simulink model "hardcode_testing_with_rate_adaptive"  (R2020b)
settings: Solver=FixedStepAuto  StartTime=0.0  StopTime=30  FixedStep=1E-3  RelTol=1e-3  EnableMultiTasking=on
undefined symbols (not defined in the file): D0, D1, D10, D11, D12, D13, D2, D3, D4, D5, D6, D7, D8, D9, PTA0, PTA1, PTA2, PTB23, PTB9, PTC16, PTC17, PTC2, PTC3, PTC4, PTD0, PTD1, PTD2, PTD3
libraries: frdmk64flib x17
settings Model: SimulationMode=external  ExtModeTrigDuration=5  Creator=Owner  LastModifiedBy=saihajgill
settings OptimizationCC: EnhancedBackFolding=on  PassReuseOutputArgsAs=Individual arguments  ZeroExternalMemoryAtStartup=off  ZeroInternalMemoryAtStartup=off  MaxStackSize=64  OptimizeBlockOrder=speed  DifferentSizesBufferReuse=on  OptimizationCustomize=off  EfficientTunableParamExpr=on
settings DebuggingCC: ParameterTunabilityLossMsg=error
settings HardwareCC: ProdBitPerPointer=32  ProdBitPerSizeT=32  ProdBitPerPtrDiffT=32  ProdLargestAtomicInteger=Long  ProdLargestAtomicFloat=Double  ProdWordSize=32  ProdHWDeviceType=ARM Compatible->ARM Cortex  UseEmbeddedCoderFeatures=off
settings SFSimCC: MATLABDynamicMemAlloc=off
settings RTWCC: Description=Embedded Coder  SystemTargetFile=ert.tlc  HardwareBoard=NXP FRDM-K64F  TLCOptions="-aInlineSetEventsForThisBaseRateFcn=TLC_FALSE -aSuppressMultiTaskScheduler=TLC_FALSE  -aRateBasedStepFcn=0"  TemplateMakefile=ert_default_tmf  Toolchain=GNU Tools for ARM Embedded Processors
settings CodeAppCC: ForceParamTrailComments=on  IgnoreCustomStorageClasses=off  OperatorAnnotations=on  SimulinkDataObjDesc=on  SFDataObjDesc=on  InsertBlockDesc=on
settings ERTTargetCC: SupportNonInlinedSFcns=on  ExtModeTransport=4  ExtModeMexFile=sendToCommService

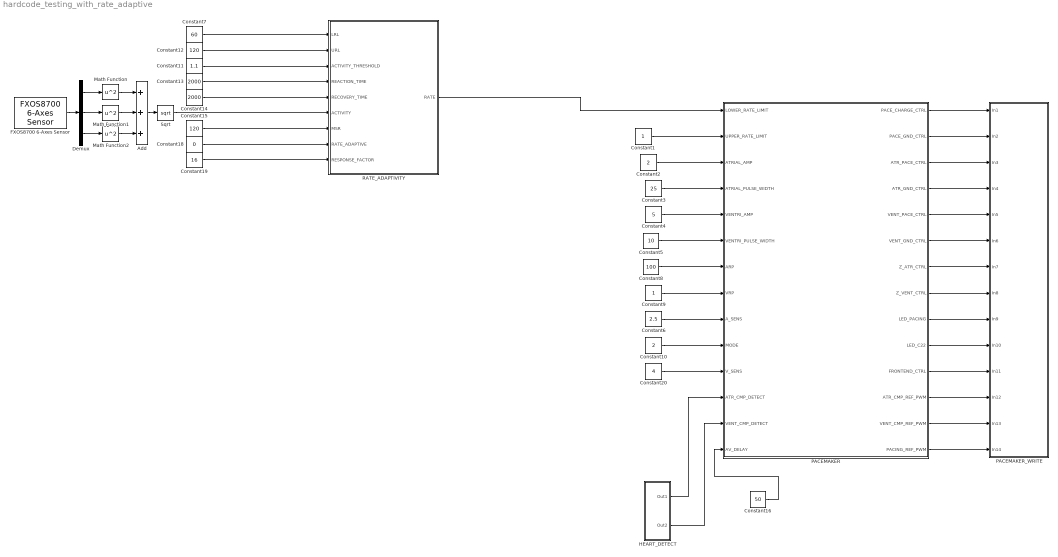
== system hardcode_testing_with_rate_adaptive ==
  Add : Sum  Inputs=+++
  Constant1 : Constant
  Constant10 : Constant  Value=2
  Constant11 : Constant  Value=1.1
  Constant12 : Constant  Value=120
  Constant13 : Constant  Value=2000
  Constant14 : Constant  Value=2000
  Constant15 : Constant  Value=120
  Constant16 : Constant  Value=50
  Constant18 : Constant  Value=0
  Constant19 : Constant  Value=16
  Constant2 : Constant  Value=2
  Constant20 : Constant  Value=4
  Constant3 : Constant  Value=25
  Constant4 : Constant  Value=5
  Constant5 : Constant  Value=10
  Constant6 : Constant  Value=2.5
  Constant7 : Constant  Value=60
  Constant8 : Constant  Value=100
  Constant9 : Constant
  Demux : Demux  Outputs=3
  FXOS8700 6-Axes Sensor : frdmk64flib/FXOS8700 6-Axes Sensor  Activesensor=Accelerometer only  ODR=800Hz  HybridODR=400Hz  Accelfullrange=-4g to +4g  SampleTime=-1
  HEART_DETECT : Subsystem
  Math Function : Math  Operator=square  SaturateOnIntegerOverflow=on
  Math Function1 : Math  Operator=square  SaturateOnIntegerOverflow=on
  Math Function2 : Math  Operator=square  SaturateOnIntegerOverflow=on
  PACEMAKER : Stateflow chart  TreatAsAtomicUnit=on
  PACEMAKER_WRITE : Subsystem
  RATE_ADAPTIVITY : Stateflow chart  TreatAsAtomicUnit=on
  Sqrt : Sqrt  SaturateOnIntegerOverflow=on
  wires:
  Constant1/1 -> PACEMAKER/2(UPPER_RATE_LIMIT)
  Constant2/1 -> PACEMAKER/3(ATRIAL_AMP)
  Constant3/1 -> PACEMAKER/4(ATRIAL_PULSE_WIDTH)
  Constant4/1 -> PACEMAKER/5(VENTRI_AMP)
  Constant5/1 -> PACEMAKER/6(VENTRI_PULSE_WIDTH)
  Constant8/1 -> PACEMAKER/7(ARP)
  Constant9/1 -> PACEMAKER/8(VRP)
  Constant10/1 -> PACEMAKER/10(MODE)
  Constant6/1 -> PACEMAKER/9(A_SENS)
  PACEMAKER/1(PACE_CHARGE_CTRL) -> PACEMAKER_WRITE/1(In1)
  PACEMAKER/2(PACE_GND_CTRL) -> PACEMAKER_WRITE/2(In2)
  PACEMAKER/3(ATR_PACE_CTRL) -> PACEMAKER_WRITE/3(In3)
  PACEMAKER/4(ATR_GND_CTRL) -> PACEMAKER_WRITE/4(In4)
  PACEMAKER/5(VENT_PACE_CTRL) -> PACEMAKER_WRITE/5(In5)
  PACEMAKER/6(VENT_GND_CTRL) -> PACEMAKER_WRITE/6(In6)
  PACEMAKER/7(Z_ATR_CTRL) -> PACEMAKER_WRITE/7(In7)
  PACEMAKER/8(Z_VENT_CTRL) -> PACEMAKER_WRITE/8(In8)
  PACEMAKER/9(LED_PACING) -> PACEMAKER_WRITE/9(In9)
  PACEMAKER/10(LED_C22) -> PACEMAKER_WRITE/10(In10)
  PACEMAKER/11(FRONTEND_CTRL) -> PACEMAKER_WRITE/11(In11)
  PACEMAKER/12(ATR_CMP_REF_PWM) -> PACEMAKER_WRITE/12(In12)
  PACEMAKER/13(VENT_CMP_REF_PWM) -> PACEMAKER_WRITE/13(In13)
  PACEMAKER/14(PACING_REF_PWM) -> PACEMAKER_WRITE/14(In14)
  HEART_DETECT/1(Out1) -> PACEMAKER/12(ATR_CMP_DETECT)
  HEART_DETECT/2(Out2) -> PACEMAKER/13(VENT_CMP_DETECT)
  Demux/2 -> Math Function1/1
  Constant15/1 -> RATE_ADAPTIVITY/7(MSR)
  Constant12/1 -> RATE_ADAPTIVITY/2(URL)
  Constant19/1 -> RATE_ADAPTIVITY/9(RESPONSE_FACTOR)
  Add/1 -> Sqrt/1
  Demux/3 -> Math Function2/1
  Constant13/1 -> RATE_ADAPTIVITY/4(REACTION_TIME)
  Constant18/1 -> RATE_ADAPTIVITY/8(RATE_ADAPTIVE)
  FXOS8700 6-Axes Sensor/1 -> Demux/1
  Math Function1/1 -> Add/2
  Constant14/1 -> RATE_ADAPTIVITY/5(RECOVERY_TIME)
  Demux/1 -> Math Function/1
  Constant7/1 -> RATE_ADAPTIVITY/1(LRL)
  Math Function2/1 -> Add/3
  Constant11/1 -> RATE_ADAPTIVITY/3(ACTIVITY_THRESHOLD)
  Math Function/1 -> Add/1
  Sqrt/1 -> RATE_ADAPTIVITY/6(ACTIVITY)
  Constant16/1 -> PACEMAKER/14(AV_DELAY)
  Constant20/1 -> PACEMAKER/11(V_SENS)
  RATE_ADAPTIVITY/1(RATE) -> PACEMAKER/1(LOWER_RATE_LIMIT)

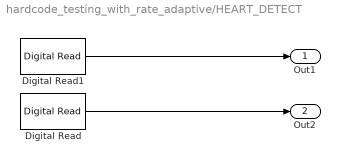
== system hardcode_testing_with_rate_adaptive/HEART_DETECT ==
  Digital Read : frdmk64flib/Digital Read  Whichpin=PTC17 (D1)  SampleTime=-1
  Digital Read1 : frdmk64flib/Digital Read  Whichpin=PTC16 (D0)  SampleTime=-1
  Out1 : Outport
  Out2 : Outport  Port=2
  wires:
  Digital Read/1 -> Out2/1
  Digital Read1/1 -> Out1/1

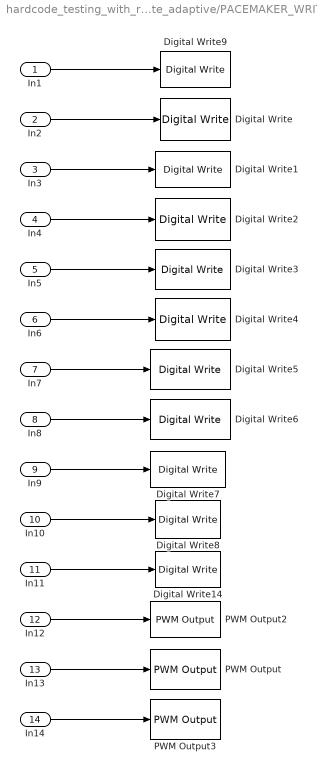
== system hardcode_testing_with_rate_adaptive/PACEMAKER_WRITE ==
  In1 : Inport
  In2 : Inport  Port=2
  In3 : Inport  Port=3
  In4 : Inport  Port=4
  In5 : Inport  Port=5
  In6 : Inport  Port=6
  In7 : Inport  Port=7
  In8 : Inport  Port=8
  In9 : Inport  Port=9
  In10 : Inport  Port=10
  In11 : Inport  Port=11
  In12 : Inport  Port=12
  In13 : Inport  Port=13
  In14 : Inport  Port=14
  Digital Write : frdmk64flib/Digital Write  Whichpin=PTD0 (D10)
  Digital Write1 : frdmk64flib/Digital Write  Whichpin=PTA0 (D8)
  Digital Write14 : frdmk64flib/Digital Write  Whichpin=PTD1 (D13)
  Digital Write2 : frdmk64flib/Digital Write  Whichpin=PTD2 (D11)
  Digital Write3 : frdmk64flib/Digital Write  Whichpin=PTC4 (D9)
  Digital Write4 : frdmk64flib/Digital Write  Whichpin=PTD3 (D12)
  Digital Write5 : frdmk64flib/Digital Write  Whichpin=PTB23 (D4)
  Digital Write6 : frdmk64flib/Digital Write  Whichpin=PTC3 (D7)
  Digital Write7 : frdmk64flib/Digital Write  Whichpin=RED_LED
  Digital Write8 : frdmk64flib/Digital Write  Whichpin=BLUE_LED
  Digital Write9 : frdmk64flib/Digital Write  Whichpin=PTB9 (D2)
  PWM Output : frdmk64flib/PWM Output  Whichpin=PTA1 (D3)  InitialFrequency=2000  InitialDutyCycle=100
  PWM Output2 : frdmk64flib/PWM Output  Whichpin=PTC2 (D6)  InitialFrequency=2000  InitialDutyCycle=100
  PWM Output3 : frdmk64flib/PWM Output  Whichpin=PTA2 (D5)  InitialFrequency=2000  InitialDutyCycle=100
  wires:
  In10/1 -> Digital Write8/1
  In2/1 -> Digital Write/1
  In12/1 -> PWM Output2/1
  In7/1 -> Digital Write5/1
  In4/1 -> Digital Write2/1
  In8/1 -> Digital Write6/1
  In11/1 -> Digital Write14/1
  In1/1 -> Digital Write9/1
  In6/1 -> Digital Write4/1
  In9/1 -> Digital Write7/1
  In14/1 -> PWM Output3/1
  In3/1 -> Digital Write1/1
  In13/1 -> PWM Output/1
  In5/1 -> Digital Write3/1

== stateflow chart hardcode_testing_with_rate_adaptive/RATE_ADAPTIVITY ==
  state BELOW_THRESHOLD [commented out]
    ADJUSTED_BPM = LRL
  state DEFAULT [commented out]
  state ADJUSTED_BPM [commented out]
    entry:
    ADJUSTED_BPM = 13/RESPONSE_FACTOR*(ACTIVITY- ACTIVITY_THRESHOLD)+LRL
  state INIT1 [commented out]
    AVG_ACCEL = 0
    n = 0
  state MIN_RATE
    AVG_ACTIVITY = (AVG_ACTIVITY + ACTIVITY)/2
    if RATE > LRL
    RATE = RATE - (MSR-LRL)/RECOVERY_TIME
    DELAY = RECOVERY_TIME
    else
    RATE = LRL
    DELAY = 0
    end
  state TRANSITION [commented out]
  state INITIAL
    RATE = LRL
    AVG_ACTIVITY = ACTIVITY
  state RATE_ADAPTIVE_DEFAULT
  state RATE_ADAPTIVE
    ADJUSTED_RATE = (0.57*RESPONSE_FACTOR^2-1.34*RESPONSE_FACTOR+22.71)*(AVG_ACTIVITY- double(ACTIVITY_THRESHOLD))+LRL
    if ADJUSTED_RATE > MSR
    ADJUSTED_RATE = MSR
    elseif ADJUSTED_RATE < LRL
    ADJUSTED_RATE = LRL
    end
  state OFFSET
    AVG_ACTIVITY = (AVG_ACTIVITY + ACTIVITY)/2
    if RATE > ADJUSTED_RATE
    RATE = RATE - (MSR-LRL)/RECOVERY_TIME
    DELAY = RECOVERY_TIME
    elseif RATE < ADJUSTED_RATE
    RATE = RATE + (MSR-LRL)/REACTION_TIME
    DELAY = REACTION_TIME
    end
  state INIT [commented out]
    ADJUSTED_BPM = LRL
  state MIN_BPM [commented out]
    ADJUSTED_BPM = LRL
  state SAME_BPM [commented out]
    %no change in bpm
  state UP_BPM [commented out]
    ADJUSTED_BPM =ADJUSTED_BPM + OFFSET
  state MAX_BPM [commented out]
    ADJUSTED_BPM = URL
  state DOWN_BPM [commented out]
    ADJUSTED_BPM = ADJUSTED_BPM - OFFSET
  DEFAULT -> BELOW_THRESHOLD [commented out] : [n>= REACTION_TIME && AVG_ACCEL <= ACTIVITY_THRESHOLD]
  BELOW_THRESHOLD -> DEFAULT [commented out] : {n=1}
  DEFAULT -> DEFAULT [commented out] : [after(1,msec)]{n = n+1, PREV_ACCEL = AVG_ACCEL, AVG_ACCEL = (AVG_ACCEL + CURR_ACCEL)/2}
  (default) -> INIT1 [commented out]
  DEFAULT -> ADJUSTED_BPM [commented out] : [n>= REACTION_TIME && AVG_ACCEL > PREV_ACCEL && AVG_ACCEL >ACTIVITY_THRESHOLD]
  INIT1 -> DEFAULT [commented out]
  DEFAULT -> ADJUSTED_BPM [commented out] : [n>= RECOVERY_TIME && AVG_ACCEL < PREV_ACCEL && AVG_ACCEL > ACTIVITY_THRESHOLD]
  ADJUSTED_BPM -> TRANSITION [commented out] : {n=1}
  TRANSITION -> DEFAULT [commented out] : [BPM >= URL]{BPM = URL, BPM_PREV = BPM}
  TRANSITION -> DEFAULT [commented out] : [BPM >= MSR]{BPM = MSR, BPM_PREV = BPM}
  MIN_RATE -> RATE_ADAPTIVE [order 1] : [n>= DELAY && AVG_ACTIVITY>=ACTIVITY_THRESHOLD]
  MIN_RATE -> MIN_RATE [order 2] : after(1,msec){n=n+1}
  MIN_RATE -> INITIAL [order 3] : [RATE_ADAPTIVE == 0 && n>=DELAY]
  RATE_ADAPTIVE_DEFAULT -> MIN_RATE [order 2] : [AVG_ACTIVITY < ACTIVITY_THRESHOLD]{n=0}
  (default) -> INITIAL
  INITIAL -> RATE_ADAPTIVE_DEFAULT : [RATE_ADAPTIVE == 1]{ADJUSTED_RATE = RATE}
  RATE_ADAPTIVE_DEFAULT -> RATE_ADAPTIVE [order 1] : [AVG_ACTIVITY>= ACTIVITY_THRESHOLD]
  OFFSET -> RATE_ADAPTIVE_DEFAULT [order 1] : [n>=DELAY]
  RATE_ADAPTIVE -> OFFSET : {n=0, AVG_ACTIVITY = ACTIVITY}
  UP_BPM -> SAME_BPM [commented out] : [RATE_ADAPTIVITY == 1 && CUR_ACCEL < ACTIVITY_THRESHOLD && after(REACTION_TIME, msec)]
  OFFSET -> OFFSET [order 2] : after(1, msec){n=n+1}
  MIN_BPM -> UP_BPM [commented out] : [RATE_ADAPTIVITY == 1 && CUR_ACCEL >= ACTIVITY_THRESHOLD && after(REACTION_TIME, msec)]
  (default) -> INIT [commented out]
  SAME_BPM -> UP_BPM [commented out] : [RATE_ADAPTIVITY == 1 &&CUR_ACCEL >= ACTIVITY_THRESHOLD && after(ADJUSTED_BPM, msec)]
  INIT -> MIN_BPM [commented out] : [RATE_ADAPTIVITY == 1]{OFFSET = (MSR-LRL)/RESPONSE_FACTOR}
  DOWN_BPM -> MIN_BPM [commented out] : [RATE_ADAPTIVITY == 0 && after(RECOVERY_TIME, msec) && ADJUSTED_BPM - OFFSET <= LRL]
  DOWN_BPM -> MIN_BPM [commented out] : [RATE_ADAPTIVITY == 1 && CUR_ACCEL < ACTIVITY_THRESHOLD && after(RECOVERY_TIME, msec) && ADJUSTED_BPM - OFFSET < LRL]
  UP_BPM -> MAX_BPM [commented out] : [RATE_ADAPTIVITY == 1 && CUR_ACCEL >= ACTIVITY_THRESHOLD && after(REACTION_TIME, msec) && ADJUSTED_BPM + OFFSET > URL]
  UP_BPM -> DOWN_BPM [commented out] : [RATE_ADAPTIVITY == 0]
  UP_BPM -> UP_BPM [commented out] : [RATE_ADAPTIVITY == 1 && CUR_ACCEL >= ACTIVITY_THRESHOLD && after(REACTION_TIME, msec) && ADJUSTED_BPM + OFFSET <= URL]
  SAME_BPM -> DOWN_BPM [commented out] : [RATE_ADAPTIVITY == 0]
  DOWN_BPM -> SAME_BPM [commented out] : [RATE_ADAPTIVITY == 1 && CUR_ACCEL >= ACTIVITY_THRESHOLD && after(RECOVERY_TIME, msec)]
  MAX_BPM -> DOWN_BPM [commented out] : [RATE_ADAPTIVITY == 1 && CUR_ACCEL<ACTIVITY_THRESHOLD && after(RECOVERY_TIME, msec)]
  MAX_BPM -> DOWN_BPM [commented out] : [RATE_ADAPTIVITY == 0]
  DOWN_BPM -> DOWN_BPM [commented out] : [RATE_ADAPTIVITY == 0 && after(RECOVERY_TIME, msec) && ADJUSTED_BPM - OFFSET > LRL]
  DOWN_BPM -> DOWN_BPM [commented out] : [RATE_ADAPTIVITY == 1 && CUR_ACCEL < ACTIVITY_THRESHOLD && after(RECOVERY_TIME, msec) && ADJUSTED_BPM - OFFSET > LRL]
  data: LRL input; RATE output; URL input double; ACTIVITY_THRESHOLD input double; REACTION_TIME input double; RECOVERY_TIME input double; ACTIVITY input double; MSR input; BPM_PREV local; CURRENT_BPM local; PREV_ACCEL local; n local; AVG_ACCEL local; RATE_ADAPTIVE input; RESPONSE_FACTOR input; OFFSET local; ADJUSTED_RATE local; PREV_ACTIVITY local; AVG_ACTIVITY local; DELAY local

== stateflow chart hardcode_testing_with_rate_adaptive/PACEMAKER ==
  state ATRIUM_CHARGING
    entry:
    %Sensing Circuitry
    FRONTEND_CTRL = true
    ATR_CMP_REF_PWM = 100*A_SENS/5
    %Discharging C21
    PACE_GND_CTRL = true
    VENT_PACE_CTRL = false
    Z_ATR_CTRL = false
    Z_VENT_CTRL = false
    ATR_PACE_CTRL = false
    ATR_GND_CTRL = true
    VENT_GND_CTRL = false
    %Charging C22
    ATR_PACE_CTRL = false
    VENT_PACE_CTRL = false
    PACING_REF_PWM = 100*ATRIAL_AMP/5
    PACE_CHARGE_CTRL = true
    LED_C22 = true
    exit:
    LED_C22 = false
  state VENTRICLE_CHARGING
    entry:
    %Sensing Circuitry
    FRONTEND_CTRL = true
    VENT_CMP_REF_PWM = 100*V_SENS/5
    %Discharging C21
    PACE_GND_CTRL = true
    VENT_PACE_CTRL = false
    Z_ATR_CTRL = false
    Z_VENT_CTRL = false
    ATR_PACE_CTRL = false
    ATR_GND_CTRL = false
    VENT_GND_CTRL = true
    %Charging C22
    ATR_PACE_CTRL = false
    VENT_PACE_CTRL = false
    PACING_REF_PWM = 100*VENTRI_AMP/5
    PACE_CHARGE_CTRL = true
    LED_C22 = true
    exit:
    LED_C22 = false
  state PACING_VENTRICLE
    entry:
    PACE_CHARGE_CTRL = false
    PACE_GND_CTRL = true
    ATR_PACE_CTRL = false
    ATR_GND_CTRL = false
    Z_ATR_CTRL = false
    Z_VENT_CTRL = false
    VENT_GND_CTRL = false
    VENT_PACE_CTRL = true
    LED_PACING = true
    exit:
    LED_PACING = false
  state PACING_ATRIUM
    entry:
    PACE_CHARGE_CTRL = false
    PACE_GND_CTRL = true
    ATR_PACE_CTRL = true
    ATR_GND_CTRL = false
    Z_ATR_CTRL = false
    Z_VENT_CTRL = false
    VENT_GND_CTRL = false
    VENT_PACE_CTRL = false
    LED_PACING = true
    exit:
    LED_PACING = false
  state INITIAL
    %initial state
  state CHARGING_DOO_2
    entry:
    %Discharging C21 Atrium
    PACE_GND_CTRL = true
    VENT_PACE_CTRL = false
    Z_ATR_CTRL = false
    Z_VENT_CTRL = false
    ATR_GND_CTRL = false
    ATR_PACE_CTRL = true
    VENT_GND_CTRL = false
    %Charging C22 Ventricle
    ATR_PACE_CTRL = false
    VENT_PACE_CTRL = false
    PACING_REF_PWM = 100*VENTRI_AMP/5
    PACE_CHARGE_CTRL = true
    LED_C22 = true
    exit:
    LED_C22 = false
  state CHARGING_DOO
    entry:
    %Discharging C21 Ventricle
    PACE_GND_CTRL = true
    VENT_PACE_CTRL = false
    Z_ATR_CTRL = false
    Z_VENT_CTRL = false
    ATR_GND_CTRL = false
    ATR_PACE_CTRL = false
    VENT_GND_CTRL = true
    %Charging C22 Atrium
    ATR_PACE_CTRL = false
    VENT_PACE_CTRL = false
    PACING_REF_PWM = 100*ATRIAL_AMP/5
    PACE_CHARGE_CTRL = true
    LED_C22 = true
    exit:
    LED_C22 = false
  state PACING_ATRIUM_DOO
    entry:
    PACE_CHARGE_CTRL = false
    PACE_GND_CTRL = true
    ATR_PACE_CTRL = true
    ATR_GND_CTRL = false
    Z_ATR_CTRL = false
    Z_VENT_CTRL = false
    VENT_GND_CTRL = false
    VENT_PACE_CTRL = false
    LED_PACING = true
    exit:
    LED_PACING = false
  state PACING_VENTRICLE_DOO
    entry:
    PACE_CHARGE_CTRL = false
    PACE_GND_CTRL = true
    ATR_PACE_CTRL = false
    ATR_GND_CTRL = false
    Z_ATR_CTRL = false
    Z_VENT_CTRL = false
    VENT_GND_CTRL = false
    VENT_PACE_CTRL = true
    LED_PACING = true
    exit:
    LED_PACING = false
  VENTRICLE_CHARGING -> ATRIUM_CHARGING [order 3] : [MODE == 0 || MODE == 2]
  ATRIUM_CHARGING -> VENTRICLE_CHARGING [order 3] : [MODE == 1 || MODE == 3]
  ATRIUM_CHARGING -> PACING_ATRIUM [order 1] : after(((60000/LOWER_RATE_LIMIT)-ATRIAL_PULSE_WIDTH), msec)
  VENTRICLE_CHARGING -> PACING_VENTRICLE [order 1] : after(((60000/LOWER_RATE_LIMIT)-VENTRI_PULSE_WIDTH), msec)
  INITIAL -> ATRIUM_CHARGING [order 1] : [MODE == 0 || MODE == 2]
  INITIAL -> VENTRICLE_CHARGING [order 2] : [MODE == 1 || MODE == 3]
  (default) -> INITIAL
  INITIAL -> CHARGING_DOO [order 3] : [MODE == 4]
  PACING_ATRIUM -> ATRIUM_CHARGING : after(ATRIAL_PULSE_WIDTH, msec)
  PACING_VENTRICLE -> VENTRICLE_CHARGING : after(VENTRI_PULSE_WIDTH, msec)
  VENTRICLE_CHARGING -> VENTRICLE_CHARGING [order 2] : after(VRP,msec) [MODE ==3 && VENT_CMP_DETECT == true]
  CHARGING_DOO_2 -> VENTRICLE_CHARGING [order 2] : [MODE == 1 || MODE == 3]
  CHARGING_DOO -> ATRIUM_CHARGING [order 2] : [MODE == 0 || MODE == 2]
  ATRIUM_CHARGING -> ATRIUM_CHARGING [order 2] : after(ARP,msec) [MODE == 2 && ATR_CMP_DETECT == true]
  CHARGING_DOO -> PACING_ATRIUM_DOO [order 1] : after(((60000/LOWER_RATE_LIMIT)-VENTRI_PULSE_WIDTH-AV_DELAY), msec)
  PACING_ATRIUM_DOO -> CHARGING_DOO_2 : after(ATRIAL_PULSE_WIDTH, msec)
  CHARGING_DOO_2 -> PACING_VENTRICLE_DOO [order 1] : after((AV_DELAY-ATRIAL_PULSE_WIDTH), msec)
  PACING_VENTRICLE_DOO -> CHARGING_DOO : after(VENTRI_PULSE_WIDTH, msec)
  data: PACE_CHARGE_CTRL output; PACE_GND_CTRL output; ATR_PACE_CTRL output; ATR_GND_CTRL output; VENT_PACE_CTRL output; VENT_GND_CTRL output; Z_ATR_CTRL output; Z_VENT_CTRL output; LED_PACING output; LED_C22 output; LOWER_RATE_LIMIT input; UPPER_RATE_LIMIT input; ATRIAL_AMP input; ATRIAL_PULSE_WIDTH input; VENTRI_AMP input; VENTRI_PULSE_WIDTH input; ARP input; VRP input; FRONTEND_CTRL output; ATR_CMP_REF_PWM output; VENT_CMP_REF_PWM output; PACING_REF_PWM output; A_SENS input; MODE input; V_SENS input; ATR_CMP_DETECT input; VENT_CMP_DETECT input; AV_DELAY input
